simulink model "animation_2017a"  (R2017a)
settings: Solver=VariableStepAuto  StartTime=0.0  StopTime=inf  RelTol=1e-3
libraries: vrlib x2, sharedtransform x1, aerolibanimutils x1, dspnetwork x1
settings Model: Creator=bbingham  LastModifiedBy=A01249622

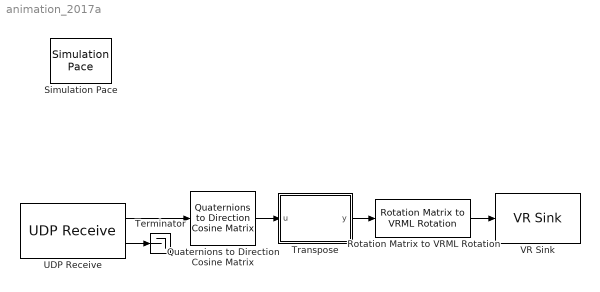
== system animation_2017a ==
  Quaternions to Direction Cosine Matrix : sharedtransform/Quaternions to  Direction Cosine Matrix
      settings: SourceProductName=Aerospace Blockset  SourceProductBaseCode=AE
  Rotation Matrix to VRML Rotation : vrlib/Utilities/Rotation Matrix to VRML Rotation  maxzero=1e-12
      settings: SourceProductName=Simulink 3D Animation  SourceProductBaseCode=VR
  Simulation Pace : aerolibanimutils/Simulation Pace  SimulationPace=1  SleepMode=MATLAB Thread  OutputPaceError=off  SampleTime=0.001
  Terminator : Terminator
  Transpose : MATLAB Function  TreatAsAtomicUnit=on
  UDP Receive : dspnetwork/UDP Receive  localURL='0.0.0.0'  localPort=12346  remoteURL='10.128.1.9'  remotePort=-1  recvBufferSize=32  dims=4  signalDatatype=double  isVarSize=off  showBlockingTime=off  blockingTime=0  sampletime=0.001  blockPlatform=[]
      settings: SourceProductName=DSP System Toolbox  SourceProductBaseCode=DS
  VR Sink : vrlib/VR Sink  InstantiateOnLoad=on  SampleTime=-1  ViewEnable=on  RemoteChange=off  RemoteView=off  FieldsWritten=Full_Model.rotation.4.1.1.double  WorldFileName=SparkFun_9DoF_Sensor_Stick.wrl  AutoView=off  VideoDimensions=[]  AllowVariableSize=off
      settings: SourceProductBaseCode=VR
  wires:
  UDP Receive/1 -> Quaternions to Direction Cosine Matrix/1
  Rotation Matrix to VRML Rotation/1 -> VR Sink/1
  Quaternions to Direction Cosine Matrix/1 -> Transpose/1(u)
  Transpose/1(y) -> Rotation Matrix to VRML Rotation/1
  UDP Receive/2 -> Terminator/1

== matlab function animation_2017a/Transpose ==
  data: u input; y output
function y = fcn(u)

y = u';
